simulink model "swing_up_bang_bang"  (R2019b)
settings: Solver=FixedStepAuto  StartTime=0.0  StopTime=25  FixedStep=0.002  RelTol=1e-3
undefined symbols (not defined in the file): Klqi_int, Klqi_state, Parameters
settings Model: Creator=Samsung  LastModifiedBy=Samsung

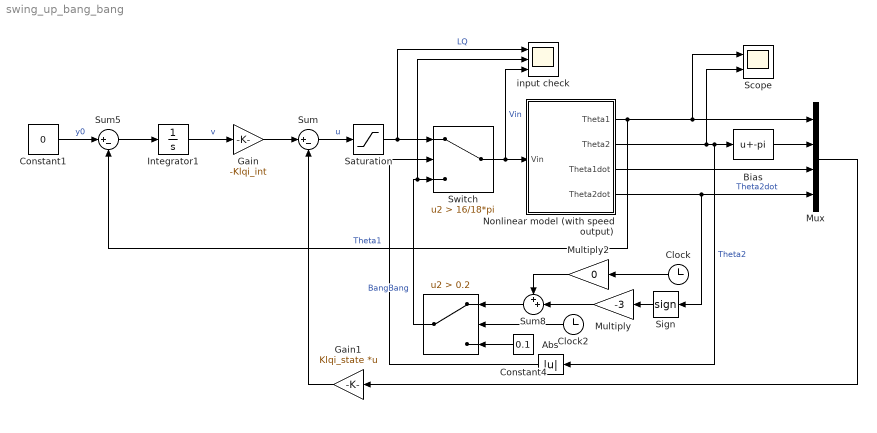
== system swing_up_bang_bang ==
  " " : Switch  Criteria=u2 > Threshold  Threshold=0.2
  Abs : Abs
  Bias : Bias  Bias=-pi
  Clock : Clock
  Clock2 : Clock
  Constant1 : Constant  Value=0
  Constant4 : Constant  Value=0.1
  Gain : Gain  Gain=-Klqi_int
  Gain1 : Gain  Gain=Klqi_state  Multiplication=Matrix(K*u)
  Integrator1 : Integrator
  Multiply : Gain  Gain=-3
  Multiply2 : Gain  Gain=0
  Mux : Mux
  Nonlinear model (with speed output) : Subsystem
  Saturation : Saturate  UpperLimit=10  LowerLimit=-10
  Scope : Scope  NumInputPorts=2
  Sign : Signum
  Sum : Sum  Inputs=|+-
  Sum5 : Sum  Inputs=|+-
  Sum8 : Sum  Inputs=++|
  Switch : Switch  Criteria=u2 > Threshold  Threshold=16/18*pi
  input check : Scope  NumInputPorts=3
  wires:
  Nonlinear model (with speed output)/1(Theta1) -> Mux/1, Scope/1, Sum5/2  "Theta1"
  Nonlinear model (with speed output)/2(Theta2) -> Scope/2, Bias/1, Abs/1  "Theta2"
  Gain1/1 -> Sum/2
  Sum/1 -> Saturation/1  "u"
  Nonlinear model (with speed output)/3(Theta1dot) -> Mux/3
  Integrator1/1 -> Gain/1  "v"
  Gain/1 -> Sum/1
  Bias/1 -> Mux/2
  Constant1/1 -> Sum5/1  "y0"
  Sum5/1 -> Integrator1/1
  Mux/1 -> Gain1/1
  Switch/1 -> input check/3, Nonlinear model (with speed output)/1(Vin)  "Vin"
  Saturation/1 -> input check/1, Switch/1  "LQ"
  Constant4/1 -> " "/3
  Nonlinear model (with speed output)/4(Theta2dot) -> Sign/1, Mux/4  "Theta2dot"
  Clock2/1 -> " "/2
  " "/1 -> input check/2, Switch/3  "BangBang"
  Sign/1 -> Multiply/1
  Sum8/1 -> " "/1
  Multiply/1 -> Sum8/2
  Clock/1 -> Multiply2/1
  Multiply2/1 -> Sum8/1
  Abs/1 -> Switch/2

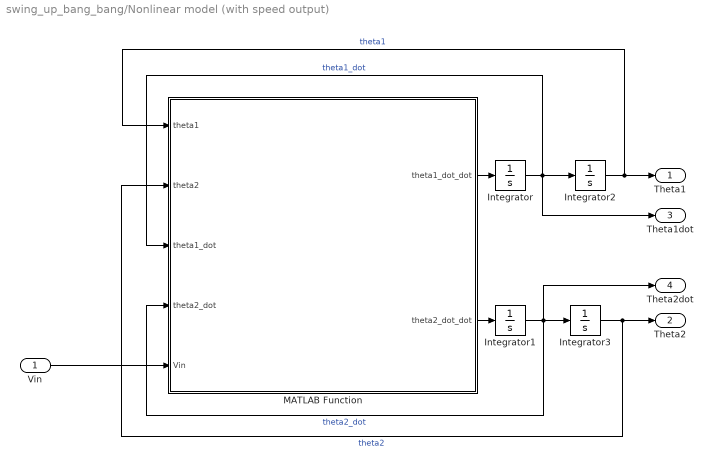
== system swing_up_bang_bang/Nonlinear model (with speed output) ==
  Vin : Inport
  Integrator{,1..3} (4 alike) : Integrator
  MATLAB Function : MATLAB Function  TreatAsAtomicUnit=on  mask{Pars=Parameters}
      mask prompts: Pars "Struct containing model parameters"
  Theta1 : Outport
  Theta2 : Outport  Port=2
  Theta1dot : Outport  Port=3
  Theta2dot : Outport  Port=4
  wires:
  Integrator/1 -> Theta1dot/1, MATLAB Function/3(theta1_dot), Integrator2/1  "theta1_dot"
  Integrator1/1 -> Theta2dot/1, MATLAB Function/4(theta2_dot), Integrator3/1  "theta2_dot"
  MATLAB Function/1(theta1_dot_dot) -> Integrator/1
  Integrator3/1 -> Theta2/1, MATLAB Function/2(theta2)  "theta2"
  MATLAB Function/2(theta2_dot_dot) -> Integrator1/1
  Integrator2/1 -> MATLAB Function/1(theta1), Theta1/1  "theta1"
  Vin/1 -> MATLAB Function/5(Vin)

== matlab function swing_up_bang_bang/Nonlinear model (with speed output)/MATLAB Function ==
  data: theta1 input; theta1_dot_dot output; theta2 input; theta1_dot input; theta2_dot input; Vin input; theta2_dot_dot output; Pars parameter
function [theta1_dot_dot,theta2_dot_dot] = fcn(theta1, theta2, theta1_dot, theta2_dot,Vin, Pars)

   k1 = Pars.Jeq + Pars.m2*(Pars.l1^2 + Pars.x2^2*sin(theta2)^2);
   k2 = Pars.m2*Pars.l1*Pars.x2*cos(theta2);
   k3 = 2*Pars.m2*Pars.x2^2*sin(theta2)*cos(theta2)*theta1_dot*theta2_dot - Pars.m2*Pars.l1*Pars.x2*sin(theta2)*theta2_dot^2 +Pars.Ks*theta1 - Pars.Km/Pars.Rm*Vin + (Pars.Km^2)/Pars.Rm*theta1_dot + Pars.Kf1*theta1_dot;
   k4 = Pars.m2*Pars.l1*Pars.x2*cos(theta2);
   k5 = Pars.m2*Pars.x2^2 + Pars.I2;
   k6 = - Pars.m2*Pars.x2^2*sin(theta2)*cos(theta2)*theta1_dot^2 + Pars.m2*Pars.g*Pars.x2*sin(theta2) + Pars.Kf2*theta2_dot;


theta1_dot_dot = (k2*k6 - k3*k5)/(k1*k5 - k2*k4);
theta2_dot_dot = -(k1*k6 - k3*k4)/(k1*k5 - k2*k4);
